simulink model "Example_simscape"  (R2020a)
settings: Solver=ode15s  StartTime=0.0  StopTime=t_simulation  RelTol=1e-4
values from neighbouring files (symbols this model uses):
  b = 0.003    [Example_script.m]
  L1 = 0.015    [Example_script.m]
  u_force = [ ... (first row only)    [Example_script.m]
libraries: nesl_utility x7, sm_lib x3, BeamStressLib x1
settings Model: Creator=mora  LastModifiedBy=mora
settings SolverCC: ZeroCrossControl=EnableAll  ZeroCrossAlgorithm=Adaptive
settings SFSimCC: CustomCodeUndefinedFunction=UseInterfaceOnly

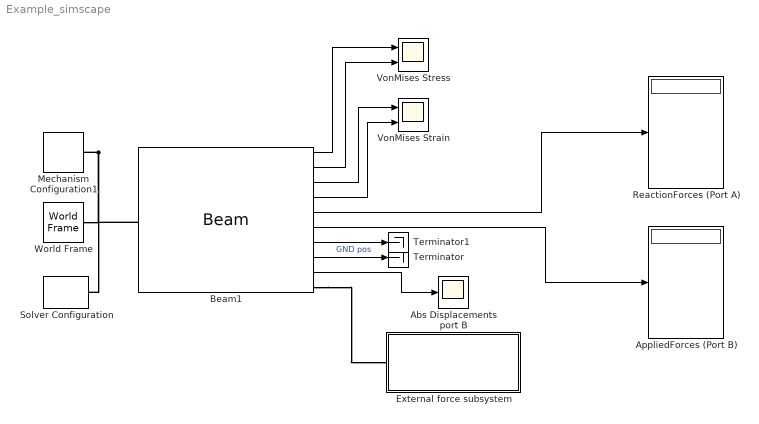
== system Example_simscape ==
  Abs Displacements port B : Scope
  AppliedForces (Port B) : Display
  Beam1 : BeamStressLib/Beam  E=E  nu=nu  rho=rho  beta=dampingConstant  L=L1  b=b  h=t  Parameter17=on  Parameter18=on  Parameter13=off  Parameter14=off  FlagPlotStress=on  TimeStartPlot=99.99  BeamID=1  Indx_BandedOrSmooth=Banded  N_elements=N_elements  BeamColor=[0.5 0.5 0.5]  Opacity=1
  External force subsystem : Subsystem
  Mechanism Configuration1 : sm_lib/Utilities/Mechanism Configuration  UniformGravity=None  GravityVector=[0 0 -9.80665]  GravityUnits=m/s^2  LinearizationDelta=0.001
  ReactionForces (Port A) : Display
  Solver Configuration : nesl_utility/Solver Configuration  PhysicalDomain=network_engine_domain  SubClassName=solver  LeftPortType=input  RightPortType=generic  Tones=[]  Harmonics=[]  SimulateNoise=off  Profile=off  UseLocalSampling=off  EnableSwitchedLinearOptims=on  FrequencyDomain=off  UseCCode=off  RelTol=0.001  AbsTol=1e-06  MinStep=1e-09  ToWorkspace=off  RevertToSquareIcSolve=off  NumHomotopyIterations=100  PhasorMode=off  PhasorModeNumHarmonics=1  DoDC=off  ResidualTolerance=1e-9  UseLocalSolver=off  LocalSolverChoice=NE_BACKWARD_EULER_ADVANCER  LocalSolverSampleTime=0.001  DoFixedCost=off  MaxNonlinIter=3  MaxModeIter=2  LinearAlgebra=auto  EquationFormulation=NE_TIME_EF  DelaysMemoryBudget=1024  AutomaticFiltering=on  FilteringTimeConstant=0.001  PartitionStorageMethod=AS_NEEDED  PartitionMemoryBudget=1024  PartitionMethod=ROBUST
  Terminator : Terminator
  Terminator1 : Terminator
  VonMises Strain : Scope  NumInputPorts=2
  VonMises Stress : Scope  NumInputPorts=2
  World Frame : sm_lib/Frames and Transforms/World Frame
  wires:
  Beam1/8 -> Terminator/1  "GND pos"
  Beam1/9 -> Abs Displacements port B/1
  Beam1/7 -> Terminator1/1
  Beam1/1 -> VonMises Stress/1
  Beam1/2 -> VonMises Stress/2
  Beam1/3 -> VonMises Strain/1
  Beam1/4 -> VonMises Strain/2
  Beam1/5 -> ReactionForces (Port A)/1
  Beam1/6 -> AppliedForces (Port B)/1
  connections:
  Mechanism Configuration1/RConn1 -- Beam1/LConn1 -- World Frame/RConn1 -- Solver Configuration/RConn1
  Beam1/RConn1 -- External force subsystem/RConn1

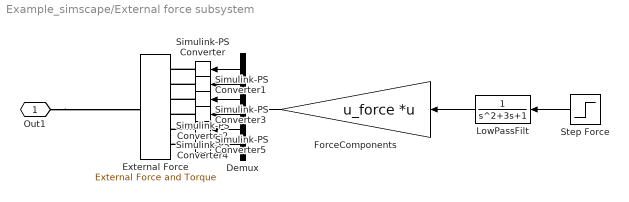
== system Example_simscape/External force subsystem ==
  Demux : Demux  Outputs=6
  External Force : sm_lib/Forces and Torques/External Force and Torque  ForceResolutionFrame=World  EnableForceX=on  EnableForceY=on  EnableForceZ=on  EnableForce=off  TorqueResolutionFrame=World  EnableTorqueX=on  EnableTorqueY=on  EnableTorqueZ=on  EnableTorque=off
  ForceComponents : Gain  Gain=u_force  Multiplication=Matrix(K*u) (u vector)
  LowPassFilt : TransferFcn  Denominator=[1 3 1]
  Simulink-PS Converter{,1..5} (6 alike) : nesl_utility/Simulink-PS Converter  PhysicalDomain=network_engine_domain  SubClassName=ps_input  LeftPortType=input  RightPortType=output  PseudoPeriodic=off  Frequencies=[]  NoiseDistribution=none  NoiseParameters=[]  Unit=1  AffineConversion=off  FilteringAndDerivatives=provide  SimscapeFilterOrder=1  InputFilterTimeConstant=0.001  UdotUserProvided=0
  Step Force : Step  SampleTime=0
  Out1 : PMIOPort  Side=Right
  wires:
  Demux/3 -> Simulink-PS Converter2/1
  Demux/1 -> Simulink-PS Converter/1
  LowPassFilt/1 -> ForceComponents/1
  Step Force/1 -> LowPassFilt/1
  Demux/2 -> Simulink-PS Converter1/1
  Demux/4 -> Simulink-PS Converter3/1
  Demux/6 -> Simulink-PS Converter5/1
  Demux/5 -> Simulink-PS Converter4/1
  ForceComponents/1 -> Demux/1
  connections:
  Simulink-PS Converter2/RConn1 -- External Force/LConn3
  Simulink-PS Converter3/RConn1 -- External Force/LConn4
  Simulink-PS Converter1/RConn1 -- External Force/LConn2
  Simulink-PS Converter/RConn1 -- External Force/LConn1
  Simulink-PS Converter4/RConn1 -- External Force/LConn5
  Simulink-PS Converter5/RConn1 -- External Force/LConn6
  Out1/RConn1 -- External Force/RConn1
